simulink model "sampleModel1478"  (R2023a)
settings: Solver=VariableStepAuto  StartTime=0.0  StopTime=10.0  RelTol=1e-3
libraries: hdlsllib x4, simulink x1
settings Model: Creator=user1  LastModifiedBy=user1

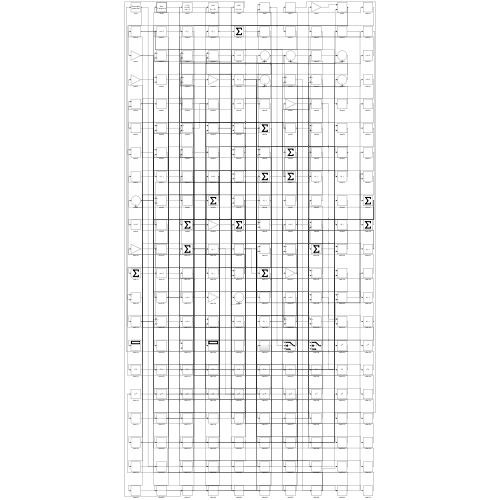
[thumbnail: Simulink's stored preview of the top-level diagram]
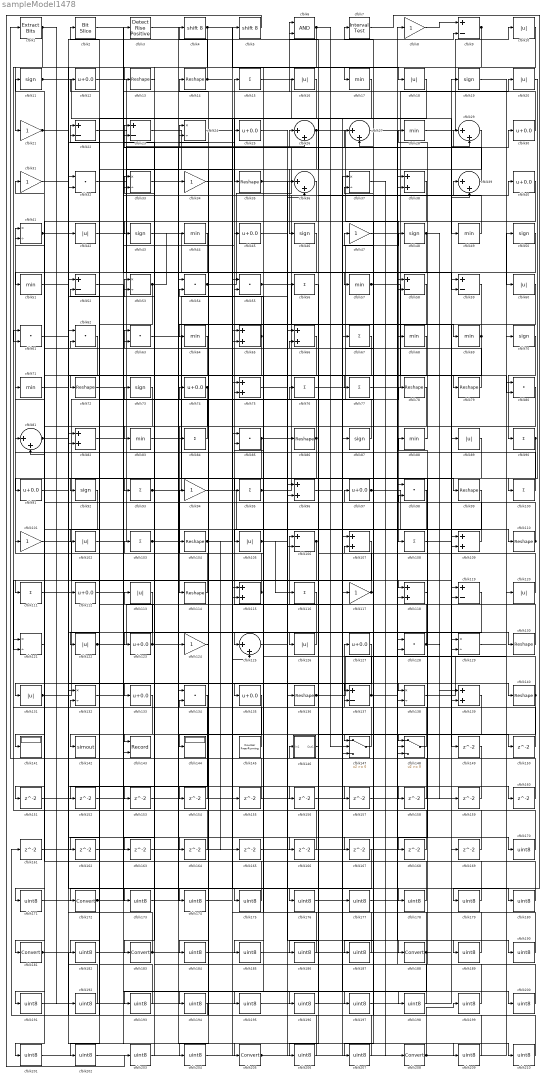
== system sampleModel1478 ==
  cfblk1 : simulink/Logic and Bit Operations/Extract Bits  bitsToExtract=Upper half  numBits=8  bitIdxRange=[0 7]  outScalingMode=Preserve fixed-point scaling
      settings: LibrarySourceBlock=|
      | hdlsllib/Logic and Bit
      | Operations/Extract Bits
  cfblk{10,16,18,20,42,60,89,102,105,113,120,122,126,131} (14 alike) : Abs  SaturateOnIntegerOverflow=off
  cfblk{15,56,67,76..77,84,90,93,95,100,103,108,111,116} (14 alike) : Sum  Inputs=+
  cfblk{8,21,31,34,47,94,101,117,124} (9 alike) : Gain
  cfblk{13..14,35,72,78..79,86,99,104,110,114,130,136,140} (14 alike) : Reshape
  cfblk{9,22..23,52,58..59,106,119,137} (9 alike) : Sum  Inputs=+-
  cfblk{38,65..66,75,82,96,107,109,115,118,139} (11 alike) : Sum
  cfblk{11,19,43,46,48,50,70,73,87,92} (10 alike) : Signum
  cfblk{12,25,30,40,45,74,91,97,112,123,127,133,135} (13 alike) : Bias  Bias=0.0  SaturateOnIntegerOverflow=off
  cfblk{24,33,37,41,53,121,129,132,138} (9 alike) : Product  Inputs=*/  RndMeth=Zero  SaturateOnIntegerOverflow=on
  cfblk{26..27,29,36,39,81,125} (7 alike) : Sum  Inputs=|++
  cfblk{32,54..55,61..63,80,85,98,128,134} (11 alike) : DotProduct  OutDataTypeStr=Inherit: Inherit via internal rule
  cfblk141 : Display
  cfblk142 : ToWorkspace  VariableName=simout  SaveFormat=Timeseries  SampleTime=-1
  cfblk143 : Record  FileSettingsInternal="{\"entries\":[{\"content\":{\"excelSettings\":{\"content\":{},\"type\":\"Streamout.ExcelSettings\"}},\"type\":\"Streamout.FileSettingStorage\",\"uuid\":\"\"}],\"packageUris\":[\"http:\\/\\/schema.mathworks.com\\/mf0\\/streamout_blocks\\/R2020a\"],\"version\":\"1.0\"}"  Layout=[1 1]  SignalsInternal="{\"entries\":[{\"content\":{\"signals\":[{\"content\":{\"blockPath\":[],\"dimensions\":[1],\"domain\":\"\",\"lineColor\":\"#a2142f\",\"plots\":[1],\"port\":1,\"signalID\":1082,\"signalName\":\"XY Graph:1\"},\"type\":\"RecordBlkView.Signal\",\"uuid\":\"\"},{\"content\":{\"blockPath\":[],\"dimensions\":[1],\"domain\":\"\",\"lineColor\":\"#139fff\",\"plots\":[1],\"port\":2,\"signalID\":1085,\"signalName\":\"XY Graph:2\"},\"type\":\"RecordBlkView.Signal\",\"uuid\":\"\"}]},\"type\":\"RecordBlkView.InputSignals\",\"uuid\":\"\"}],\"packageUris\":[\"http:\\/\\/schema.mathworks.com\\/mf0\\/streamout_blocks\\/R2020a\"],\"version\":\"1.0\"}"  VisualizationBindings="{\"xyplotplugin\":{\"info\":[{\"series\":[{\"bindingParametersList\":[{\"parameter\":\"X-Axis\",\"signalID\":1082,\"signalName\":\"XY Graph:1\"},{\"parameter\":\"Y-Axis\",\"signalID\":1085,\"signalName\":\"XY Graph:2\"}],\"seriesID\":56975}],\"subplotID\":1}]}}"  CompatibilityTag=XY  st=-1
  cfblk144 : Display
  cfblk145 : hdlsllib/Sources/Counter Free-Running  NumBits=16  tsamp=-1
  cfblk146 : Subsystem
      settings: LibrarySourceBlock=|
      | hdlsllib/Ports &
      | Subsystems/Subsystem
  cfblk147 : Switch  SaturateOnIntegerOverflow=off  InputSameDT=off
  cfblk148 : Switch  SaturateOnIntegerOverflow=off  InputSameDT=off
  cfblk{149..169} (21 alike) : Delay  SampleTime=1
  cfblk{17,28,44,49,51,57,64,68..69,71,83,88} (12 alike) : MinMax
  cfblk{170..171,173..180,182,184..187,189..204,206..207,209..210} (35 alike) : DataTypeConversion  OutDataTypeStr=uint8  SaturateOnIntegerOverflow=off  RndMeth=Floor
  cfblk{172,181,183,188,205,208} (6 alike) : DataTypeConversion  SaturateOnIntegerOverflow=off  RndMeth=Floor
  cfblk2 : hdlsllib/Logic and Bit Operations/Bit Slice  lidx=7  ridx=0
  cfblk3 : hdlsllib/Logic and Bit Operations/Detect Rise Positive  vinit=0  OutDataTypeStr=boolean
  cfblk4 : ArithShift  BitShiftNumber=8
  cfblk5 : ArithShift  BitShiftNumber=8
  cfblk6 : Logic  AllPortsSameDT=off  OutDataTypeStr=boolean
  cfblk7 : hdlsllib/Logic and Bit Operations/Interval Test  IntervalClosedRight=on  uplimit=0.5  IntervalClosedLeft=on  lowlimit=-0.5  OutDataTypeStr=boolean
  wires:
  cfblk133/1 -> cfblk142/1
  cfblk115/1 -> cfblk41/1, cfblk41/2
  cfblk128/1 -> cfblk15/1, cfblk159/1
  cfblk77/1 -> cfblk20/1
  cfblk148/1 -> cfblk127/1
  cfblk16/1 -> cfblk35/1
  cfblk102/1 -> cfblk26/2
  cfblk25/1 -> cfblk130/1
  cfblk95/1 -> cfblk39/1, cfblk118/1
  cfblk110/1 -> cfblk47/1, cfblk11/1
  cfblk73/1 -> cfblk83/1
  cfblk75/1 -> cfblk188/1
  cfblk50/1 -> cfblk51/1
  cfblk28/1 -> cfblk10/1
  cfblk17/1 -> cfblk46/1
  cfblk105/1 -> cfblk116/1, cfblk160/1, cfblk189/1
  cfblk44/1 -> cfblk72/1
  cfblk1/1 -> cfblk61/2, cfblk192/1
  cfblk54/1 -> cfblk30/1, cfblk140/1
  cfblk69/1 -> cfblk64/1, cfblk182/1
  cfblk79/1 -> cfblk31/1
  cfblk140/1 -> cfblk103/1, cfblk168/1
  cfblk126/1 -> cfblk125/1
  cfblk132/1 -> cfblk205/1
  cfblk46/1 -> cfblk131/1
  cfblk61/1 -> cfblk53/1
  cfblk42/1 -> cfblk85/1
  cfblk82/1 -> cfblk40/1
  cfblk134/1 -> cfblk172/1
  cfblk76/1 -> cfblk8/1
  cfblk4/1 -> cfblk17/1, cfblk82/2
  cfblk57/1 -> cfblk79/1, cfblk147/1
  cfblk68/1 -> cfblk77/1
  cfblk91/1 -> cfblk42/1
  cfblk122/1 -> cfblk87/1, cfblk16/1, cfblk135/1
  cfblk104/1 -> cfblk165/1, cfblk166/1
  cfblk100/1 -> cfblk81/1
  cfblk41/1 -> cfblk99/1, cfblk80/2
  cfblk32/1 -> cfblk107/1
  cfblk19/1 -> cfblk60/1
  cfblk131/1 -> cfblk34/1, cfblk138/1, cfblk156/1
  cfblk65/1 -> cfblk93/1, cfblk24/2
  cfblk119/1 -> cfblk183/1
  cfblk15/1 -> cfblk49/1
  cfblk12/1 -> cfblk86/1
  cfblk6/1 -> cfblk21/1, cfblk147/2
  cfblk93/1 -> cfblk36/2, cfblk210/1
  cfblk130/1 -> cfblk106/1
  cfblk112/1 -> cfblk45/1
  cfblk111/1 -> cfblk112/1
  cfblk23/1 -> cfblk55/1
  cfblk10/1 -> cfblk13/1
  cfblk70/1 -> cfblk90/1
  cfblk48/1 -> cfblk139/1, cfblk163/1
  cfblk20/1 -> cfblk100/1
  cfblk26/1 -> cfblk108/1, cfblk84/1
  cfblk74/1 -> cfblk114/1, cfblk91/1, cfblk81/2
  cfblk94/1 -> cfblk110/1
  cfblk55/1 -> cfblk109/1, cfblk180/1
  cfblk114/1 -> cfblk94/1
  cfblk71/1 -> cfblk109/2
  cfblk39/1 -> cfblk23/1
  cfblk136/1 -> cfblk50/1, cfblk48/1
  cfblk81/1 -> cfblk25/1, cfblk128/2, cfblk9/2
  cfblk113/1 -> cfblk123/1
  cfblk87/1 -> cfblk22/1
  cfblk88/1 -> cfblk28/1
  cfblk37/1 -> cfblk208/1
  cfblk11/1 -> cfblk67/1, cfblk115/1
  cfblk101/1 -> cfblk129/2
  cfblk27/1 -> cfblk58/1
  cfblk21/1 -> cfblk32/2, cfblk164/1
  cfblk124/1 -> cfblk104/1
  cfblk2/1 -> cfblk57/1
  cfblk147/1 -> cfblk22/2
  cfblk35/1 -> cfblk56/1, cfblk147/3, cfblk148/3
  cfblk85/1 -> cfblk133/1, cfblk143/2, cfblk138/2
  cfblk36/1 -> cfblk111/1
  cfblk72/1 -> cfblk27/1
  cfblk43/1 -> cfblk59/2
  cfblk14/1 -> cfblk4/1, cfblk18/1
  cfblk59/1 -> cfblk126/1
  cfblk89/1 -> cfblk181/1
  cfblk145/1 -> cfblk71/1
  cfblk84/1 -> cfblk2/1
  cfblk60/1 -> cfblk144/1
  cfblk138/1 -> cfblk120/1
  cfblk29/1 -> cfblk102/1
  cfblk33/1 -> cfblk69/1
  cfblk86/1 -> cfblk63/1, cfblk115/2
  cfblk64/1 -> cfblk143/1
  cfblk109/1 -> cfblk33/1
  cfblk22/1 -> cfblk125/2
  cfblk120/1 -> cfblk76/1
  cfblk30/1 -> cfblk6/1
  cfblk103/1 -> cfblk124/1, cfblk78/1, cfblk167/1
  cfblk49/1 -> cfblk24/1
  cfblk45/1 -> cfblk137/1
  cfblk137/1 -> cfblk68/1, cfblk74/1
  cfblk31/1 -> cfblk95/1
  cfblk9/1 -> cfblk43/1, cfblk105/1
  cfblk123/1 -> cfblk29/1, cfblk12/1
  cfblk97/1 -> cfblk27/2, cfblk139/2
  cfblk63/1 -> cfblk117/1
  cfblk129/1 -> cfblk70/1
  cfblk8/1 -> cfblk9/1
  cfblk106/1 -> cfblk141/1, cfblk121/2
  cfblk53/1 -> cfblk92/1, cfblk44/1
  cfblk117/1 -> cfblk107/2, cfblk187/1
  cfblk58/1 -> cfblk65/2
  cfblk118/1 -> cfblk88/1
  cfblk78/1 -> cfblk122/1
  cfblk90/1 -> cfblk148/1, cfblk148/2, cfblk118/2, cfblk152/1
  cfblk108/1 -> cfblk149/1
  cfblk149/1 -> cfblk1/1
  cfblk83/1 -> cfblk150/1
  cfblk150/1 -> cfblk53/2
  cfblk127/1 -> cfblk151/1
  cfblk151/1 -> cfblk65/1
  cfblk152/1 -> cfblk29/2
  cfblk13/1 -> cfblk153/1
  cfblk153/1 -> cfblk129/1
  cfblk80/1 -> cfblk154/1
  cfblk154/1 -> cfblk121/1
  cfblk155/1 -> cfblk32/1
  cfblk156/1 -> cfblk39/2
  cfblk125/1 -> cfblk157/1
  cfblk157/1 -> cfblk59/1
  cfblk24/1 -> cfblk158/1
  cfblk158/1 -> cfblk26/1
  cfblk159/1 -> cfblk137/2
  cfblk160/1 -> cfblk6/2
  cfblk161/1 -> cfblk54/1
  cfblk18/1 -> cfblk162/1
  cfblk162/1 -> cfblk58/2
  cfblk163/1 -> cfblk106/2
  cfblk164/1 -> cfblk33/2
  cfblk165/1 -> cfblk36/1
  cfblk166/1 -> cfblk61/1
  cfblk168/1 -> cfblk23/2
  cfblk169/1 -> cfblk55/2
  cfblk3/1 -> cfblk170/1
  cfblk170/1 -> cfblk97/1
  cfblk92/1 -> cfblk171/1
  cfblk171/1 -> cfblk3/1
  cfblk172/1 -> cfblk155/1, cfblk198/1
  cfblk135/1 -> cfblk173/1
  cfblk173/1 -> cfblk134/1
  cfblk51/1 -> cfblk174/1
  cfblk174/1 -> cfblk134/2
  cfblk38/1 -> cfblk175/1
  cfblk175/1 -> cfblk101/1
  cfblk34/1 -> cfblk176/1
  cfblk176/1 -> cfblk38/1
  cfblk177/1 -> cfblk38/2
  cfblk52/1 -> cfblk178/1
  cfblk178/1 -> cfblk14/1
  cfblk7/1 -> cfblk179/1
  cfblk179/1 -> cfblk52/1
  cfblk180/1 -> cfblk52/2
  cfblk181/1 -> cfblk169/1, cfblk209/1
  cfblk182/1 -> cfblk89/1
  cfblk183/1 -> cfblk136/1, cfblk82/1
  cfblk107/1 -> cfblk184/1
  cfblk184/1 -> cfblk119/1
  cfblk99/1 -> cfblk185/1
  cfblk185/1 -> cfblk119/2
  cfblk146/1(Out1) -> cfblk186/1
  cfblk186/1 -> cfblk85/2
  cfblk187/1 -> cfblk146/1(In1)
  cfblk188/1 -> cfblk128/1, cfblk193/1
  cfblk189/1 -> cfblk75/1
  cfblk47/1 -> cfblk190/1
  cfblk190/1 -> cfblk75/2
  cfblk62/1 -> cfblk191/1
  cfblk191/1 -> cfblk19/1
  cfblk192/1 -> cfblk62/1
  cfblk193/1 -> cfblk62/2
  cfblk66/1 -> cfblk194/1
  cfblk194/1 -> cfblk161/1
  cfblk116/1 -> cfblk195/1
  cfblk195/1 -> cfblk66/1
  cfblk139/1 -> cfblk196/1
  cfblk196/1 -> cfblk66/2
  cfblk98/1 -> cfblk197/1
  cfblk197/1 -> cfblk7/1
  cfblk198/1 -> cfblk98/1
  cfblk199/1 -> cfblk98/2
  cfblk96/1 -> cfblk200/1
  cfblk200/1 -> cfblk113/1
  cfblk121/1 -> cfblk201/1
  cfblk201/1 -> cfblk96/1
  cfblk167/1 -> cfblk202/1
  cfblk202/1 -> cfblk96/2
  cfblk5/1 -> cfblk203/1
  cfblk203/1 -> cfblk63/2
  cfblk67/1 -> cfblk204/1
  cfblk204/1 -> cfblk5/1
  cfblk205/1 -> cfblk177/1, cfblk80/1
  cfblk56/1 -> cfblk206/1
  cfblk206/1 -> cfblk132/1
  cfblk40/1 -> cfblk207/1
  cfblk207/1 -> cfblk132/2
  cfblk208/1 -> cfblk199/1, cfblk54/2, cfblk73/1
  cfblk209/1 -> cfblk37/1
  cfblk210/1 -> cfblk37/2

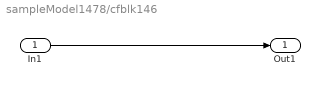
== system sampleModel1478/cfblk146 ==
  In1 : Inport
  Out1 : Outport
  wires:
  In1/1 -> Out1/1
